simulink subsystem "virtual_plant"  (R2022b)
settings: Solver=VariableStepAuto  StartTime=0.0  StopTime=10.0  RelTol=1e-3
model mask{L=0, K_m=0, J_pend=0, b=0, V_s=0, R=0, K_pend=0, K_sin=0, K_g=0, linear_mode=Linear}
  mask prompts: L "Inductance (L)"; K_m "Motor Coefficient (K_m)"; J_pend "Rotor/Pendulum Intertial (J_pend)"; b "Friction Coefficient (b)"; V_s "Source Votage (V_s)"; R "Resistance (R)"; K_pend "Pendulum On/Off (K_pend)"; K_sin "Pendulum Linearization (K_sin)"; K_g "Pendulum Coefficient (K_g)"; linear_mode "Linear/Nonlinear"
libraries: simulink x1
settings Model: Creator=Alex Zhen  LastModifiedBy=Alex Zhen

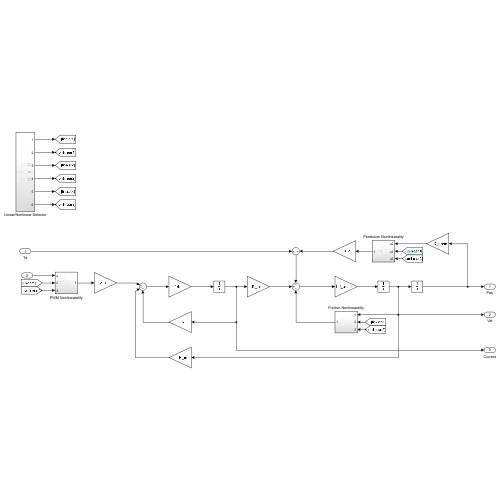
[thumbnail: Simulink's stored preview of the top-level diagram]
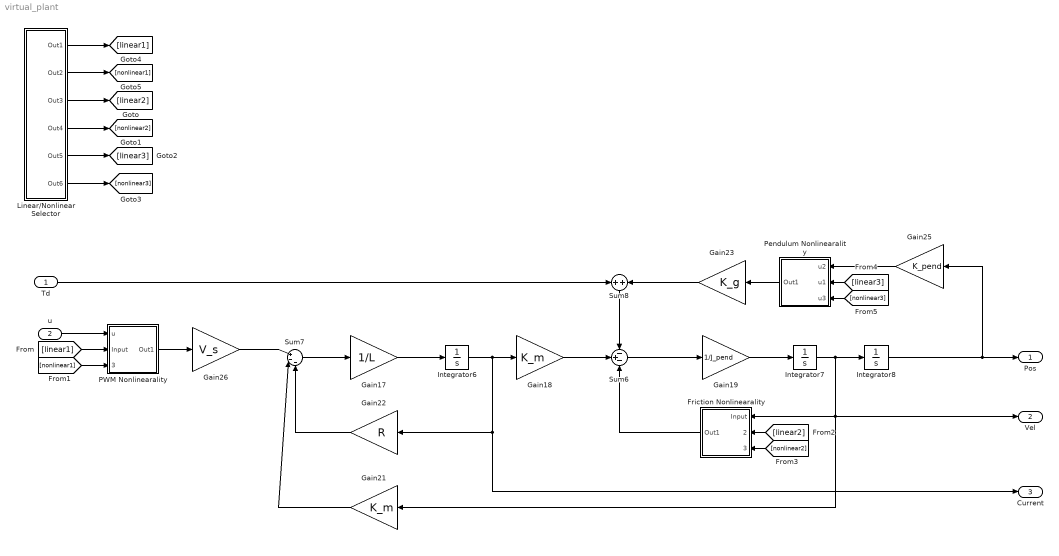
== system virtual_plant ==
  Td : Inport
  u : Inport  Port=2
  Friction Nonlinearality : Subsystem
  Gain17 : Gain  Gain=1/L
  Gain18 : Gain  Gain=K_m
  Gain19 : Gain  Gain=1/J_pend
  Gain21 : Gain  Gain=K_m
  Gain22 : Gain  Gain=R
  Gain23 : Gain  Gain=K_g
  Gain25 : Gain  Gain=K_pend
  Gain26 : Gain  Gain=V_s
  Integrator6 : Integrator
  Integrator7 : Integrator
  Integrator8 : Integrator
  Linear/Nonlinear Selector : Subsystem
  PWM Nonlinearality : Subsystem
  Pendulum Nonlinearality : Subsystem
  Sum6 : Sum  Inputs=-+-
  Sum7 : Sum  Inputs=|+--
  Sum8 : Sum
  Pos : Outport
  Vel : Outport  Port=2
  Current : Outport  Port=3
  wires:
  Sum8/1 -> Sum6/1
  Gain17/1 -> Integrator6/1
  Gain23/1 -> Sum8/2
  Gain21/1 -> Sum7/2
  Sum6/1 -> Gain19/1
  Gain26/1 -> Sum7/1
  Integrator6/1 -> Current/1, Gain22/1, Gain18/1
  Gain22/1 -> Sum7/3
  Td/1 -> Sum8/1
  Integrator7/1 -> Gain21/1, Vel/1, Friction Nonlinearality/1(Input), Integrator8/1
  Gain19/1 -> Integrator7/1
  Sum7/1 -> Gain17/1
  Gain18/1 -> Sum6/2
  Integrator8/1 -> Gain25/1, Pos/1
  u/1 -> PWM Nonlinearality/1(u)
  PWM Nonlinearality/1(Out1) -> Gain26/1
  Gain25/1 -> Pendulum Nonlinearality/1(u2)
  Pendulum Nonlinearality/1(Out1) -> Gain23/1
  Friction Nonlinearality/1(Out1) -> Sum6/3
  [linear1] -> PWM Nonlinearality/2(Input)
  [nonlinear1] -> PWM Nonlinearality/3(Input1)
  [nonlinear3] -> Pendulum Nonlinearality/3(u3)
  [linear3] -> Pendulum Nonlinearality/2(u1)
  [linear2] -> Friction Nonlinearality/2(Input1)
  [nonlinear2] -> Friction Nonlinearality/3(Input2)
  Linear/Nonlinear Selector/1(Out1) -> [linear1]
  Linear/Nonlinear Selector/2(Out2) -> [nonlinear1]
  Linear/Nonlinear Selector/3(Out3) -> [linear2]
  Linear/Nonlinear Selector/4(Out4) -> [nonlinear2]
  Linear/Nonlinear Selector/5(Out5) -> [linear3]
  Linear/Nonlinear Selector/6(Out6) -> [nonlinear3]

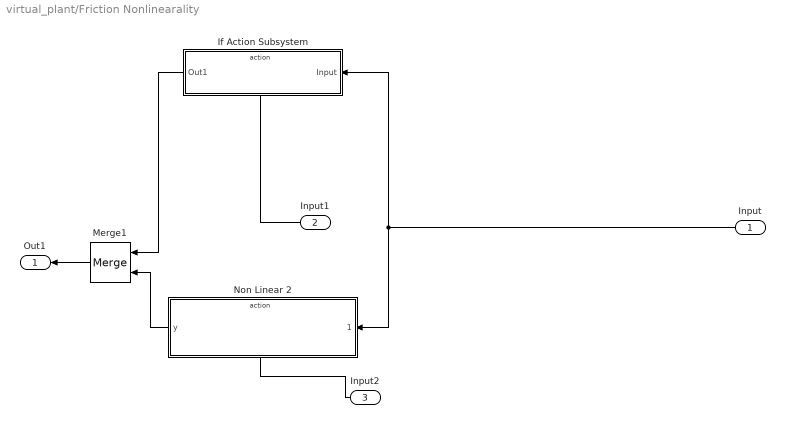
== system virtual_plant/Friction Nonlinearality ==
  Input : Inport
  Input1 : Inport  Port=2
  Input2 : Inport  Port=3
  If Action Subsystem : Subsystem  TreatAsAtomicUnit=on
  Merge1 : Merge
  Non Linear 2 : Subsystem  TreatAsAtomicUnit=on
  Out1 : Outport
  wires:
  Non Linear 2/1(y) -> Merge1/2
  If Action Subsystem/1(Out1) -> Merge1/1
  Input2/1 -> Non Linear 2/Action
  Input1/1 -> If Action Subsystem/Action
  Merge1/1 -> Out1/1
  Input/1 -> If Action Subsystem/1(Input), Non Linear 2/1(" ")

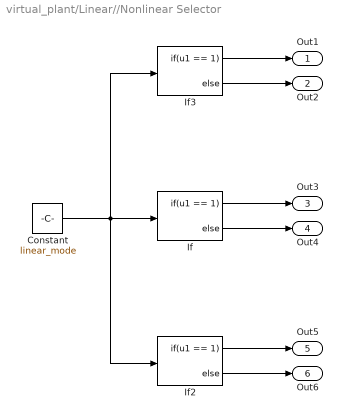
== system virtual_plant/Linear//Nonlinear Selector ==
  Constant : Constant  Value=linear_mode
  If : If  IfExpression=u1 == 1
  If2 : If  IfExpression=u1 == 1
  If3 : If  IfExpression=u1 == 1
  Out1 : Outport
  Out2 : Outport  Port=2
  Out3 : Outport  Port=3
  Out4 : Outport  Port=4
  Out5 : Outport  Port=5
  Out6 : Outport  Port=6
  wires:
  Constant/1 -> If2/1, If/1, If3/1
  If3/2 -> Out2/1
  If3/1 -> Out1/1
  If2/1 -> Out5/1
  If2/2 -> Out6/1
  If/1 -> Out3/1
  If/2 -> Out4/1

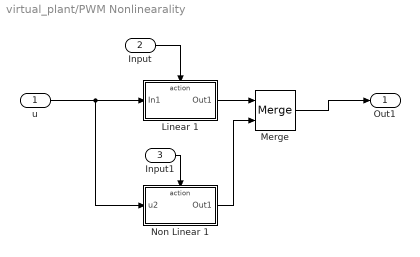
== system virtual_plant/PWM Nonlinearality ==
  u : Inport
  Input : Inport  Port=2
  Input1 : Inport  Port=3
  Linear 1 : Subsystem  TreatAsAtomicUnit=on
  Merge : Merge
  Non Linear 1 : Subsystem  TreatAsAtomicUnit=on
  Out1 : Outport
  wires:
  Non Linear 1/1(Out1) -> Merge/2
  u/1 -> Linear 1/1(In1), Non Linear 1/1(u2)
  Input1/1 -> Non Linear 1/Action
  Linear 1/1(Out1) -> Merge/1
  Input/1 -> Linear 1/Action
  Merge/1 -> Out1/1

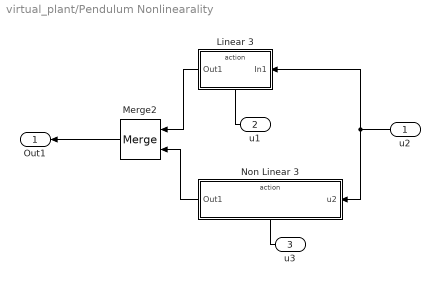
== system virtual_plant/Pendulum Nonlinearality ==
  u2 : Inport
  u1 : Inport  Port=2
  u3 : Inport  Port=3
  Linear 3 : Subsystem  TreatAsAtomicUnit=on
  Merge2 : Merge
  Non Linear 3 : Subsystem  TreatAsAtomicUnit=on
  Out1 : Outport
  wires:
  u1/1 -> Linear 3/Action
  Non Linear 3/1(Out1) -> Merge2/2
  Linear 3/1(Out1) -> Merge2/1
  u3/1 -> Non Linear 3/Action
  u2/1 -> Non Linear 3/1(u2), Linear 3/1(In1)
  Merge2/1 -> Out1/1

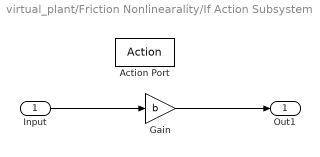
== system virtual_plant/Friction Nonlinearality/If Action Subsystem ==
  Input : Inport
  Action Port : ActionPort
  Gain : Gain  Gain=b
  Out1 : Outport
  wires:
  Input/1 -> Gain/1
  Gain/1 -> Out1/1

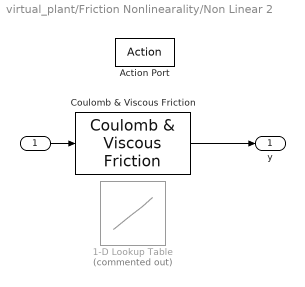
== system virtual_plant/Friction Nonlinearality/Non Linear 2 ==
  " " : Inport
  Action Port : ActionPort
  1-D Lookup Table : Lookup_n-D  Commented=on  NumberOfTableDimensions=1  BreakpointsForDimension1="[-600 -480.02 -360.04 -240.06 -120.08 -0.1 0 0.1000  120.0800  240.0600  360.0400  480.0200  600.0000]"  Table="[ -0.004 -0.0028 -0.0018 -0.0011 -0.0006 -0.0004 0 0.0004    0.0006    0.0011    0.0018    0.0028    0.0040]"  DiagnosticForOutOfRangeInput=Warning  InternalRulePriority=Speed  RndMeth=Simplest
  Coulomb & Viscous Friction : simulink/Discontinuities/Coulomb & Viscous Friction  offset=Friction_static  gain=b
  y : Outport
  wires:
  Coulomb & Viscous Friction/1 -> y/1
  " "/1 -> Coulomb & Viscous Friction/1

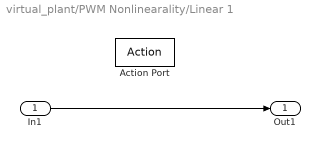
== system virtual_plant/PWM Nonlinearality/Linear 1 ==
  In1 : Inport
  Action Port : ActionPort
  Out1 : Outport
  wires:
  In1/1 -> Out1/1

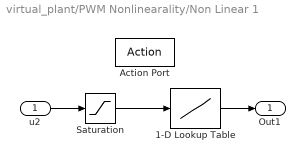
== system virtual_plant/PWM Nonlinearality/Non Linear 1 ==
  u2 : Inport
  Action Port : ActionPort
  1-D Lookup Table : Lookup_n-D  NumberOfTableDimensions=1  BreakpointsForDimension1=[-1,-0.96,-0.1,-0.06,-0.04,0,0.04,0.06,0.1,0.96,1]  Table=[-10.8,-10.8,-2,-1,-0,0,0,1,2,10.8,10.8]/V_s  InternalRulePriority=Speed  RndMeth=Simplest
  Saturation : Saturate  UpperLimit=1  LowerLimit=-1
  Out1 : Outport
  wires:
  1-D Lookup Table/1 -> Out1/1
  Saturation/1 -> 1-D Lookup Table/1
  u2/1 -> Saturation/1

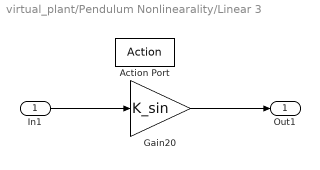
== system virtual_plant/Pendulum Nonlinearality/Linear 3 ==
  In1 : Inport
  Action Port : ActionPort
  Gain20 : Gain  Gain=K_sin
  Out1 : Outport
  wires:
  Gain20/1 -> Out1/1
  In1/1 -> Gain20/1

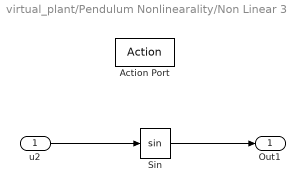
== system virtual_plant/Pendulum Nonlinearality/Non Linear 3 ==
  u2 : Inport
  Action Port : ActionPort
  Sin : Trigonometry
  Out1 : Outport
  wires:
  Sin/1 -> Out1/1
  u2/1 -> Sin/1
